simulink model "SERWO1"  (R2015b)
settings: Solver=ode1  StartTime=0.0  StopTime=Inf  FixedStep=0.001  RelTol=1e-3
PostLoadFcn:
  | , if any(exist('dsrtsu_mdlpostloadfcn', 'file') == [2, 3, 6]), try dsrtsu_mdlpostloadfcn('Execute', bdroot); catch fprintf('Error in PostLoadFcn (dsrtsu_mdlpostloadfcn) for model "%s":\n %s\n', bdroot, lasterr); end, end,
libraries: simulink x12, rtilib1104 x9
settings Model: DSRTSU_INTERNAL_RTI_VER=460  DSRTSU_INTERNAL_RTI_TYPE=rti1104  DSRTSU_INTERNAL_RTIFPGA=50  Creator=k16p800b  LastModifiedBy=lukas
settings DataIOCC: SaveFormat=Array
settings OptimizationCC: BlockReduction=off  OptimizeBlockIOStorage=off  BufferReuse=off  GlobalBufferReuse=off  ExpressionFolding=off  LocalBlockOutputs=off
settings HardwareCC: ProdBitPerPointer=32  ProdLargestAtomicFloat=None  ProdEndianess=BigEndian  ProdWordSize=32  ProdHWDeviceType=Generic->Custom  TargetIntDivRoundTo=Zero  TargetEndianess=BigEndian  TargetHWDeviceType=Generic->Custom
settings RTWCC: SystemTargetFile=rti1104.tlc  MakeCommand=make_rti  TemplateMakefile=rti1104.tmf  Description=dSPACE DS1104 Hardware Platform
settings STFCustomTargetCC: ParMdlRefBuildCompliant=on  ConcurrentExecutionCompliant=off  CPPClassGenCompliant=off  SystemTargetFile=rti1104.tlc
settings GRTTargetCC: CompOptLevelCompliant=off  ConcurrentExecutionCompliant=off  GeneratePreprocessorConditionals=Disable all  CombineOutputUpdateFcns=off  MatFileLogging=off  CPPClassGenCompliant=off  GRTInterface=on  UseToolchainInfoCompliant=off  ExtModeMexFile=noextcomm
settings ConfigComp: CovModelRefEnable=Off

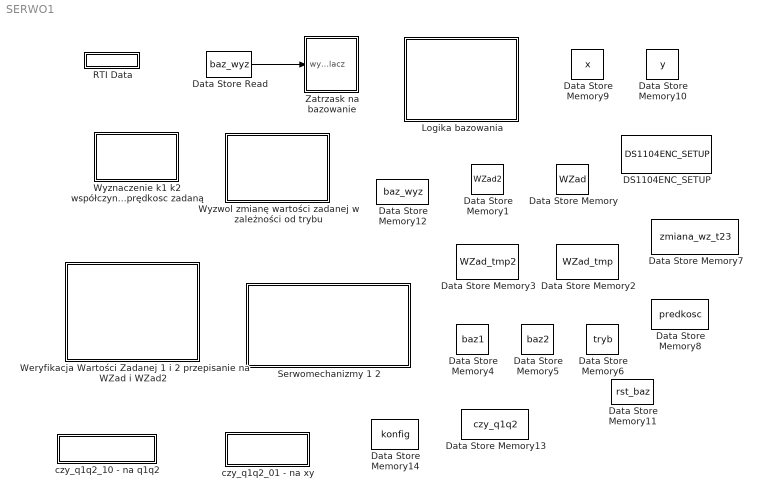
== system SERWO1 ==
  DS1104ENC_SETUP : rtilib1104/DS1104 MASTER PPC/DS1104ENC_SETUP  Reserved1=[]  Reserved2=[]  Reserved3=[]  Reserved4=[]  DialogFcn=gui1104enc_setup  UnitName={'DS1104ENC_SETUP'}  UnitValues={ [] }  DSProperties=struct('RTI',struct('Version',uint32(1),'BlockType',struct('isSLSource',uint8(0),'isSLSink',uint8(0),'isHWSource',uint8(0),'isHWSink',uint8(0),'isSetup',uint8(0),'isInline',uint8(1),'isNonInline',uint8(0),'isInterrupt',uint8(0),'isChannelwise',uint8(0)),'IOBoardType','DS1104MASTER','UnitType','ENC','Identifier','ENCSETUP','DialogType','ML','BlockSet','NONE','SlaveProcessor','NONE'))
      settings: SignalType=[0 0]
  Data Store Memory : DataStoreMemory  DataStoreName=WZad  ReadBeforeWriteMsg=warning  WriteAfterWriteMsg=warning  WriteAfterReadMsg=warning
      settings: RTWStateStorageClass=ExportedGlobal
  Data Store Memory1 : DataStoreMemory  DataStoreName=WZad2  ReadBeforeWriteMsg=warning  WriteAfterWriteMsg=warning  WriteAfterReadMsg=warning
      settings: RTWStateStorageClass=ExportedGlobal
  Data Store Memory10 : DataStoreMemory  DataStoreName=y  ReadBeforeWriteMsg=warning  WriteAfterWriteMsg=warning  WriteAfterReadMsg=warning
  Data Store Memory11 : DataStoreMemory  DataStoreName=rst_baz  ReadBeforeWriteMsg=warning  WriteAfterWriteMsg=warning  WriteAfterReadMsg=warning
  Data Store Memory12 : DataStoreMemory  DataStoreName=baz_wyz  ReadBeforeWriteMsg=warning  WriteAfterWriteMsg=warning  WriteAfterReadMsg=warning
  Data Store Memory13 : DataStoreMemory  DataStoreName=czy_q1q2  ReadBeforeWriteMsg=warning  WriteAfterWriteMsg=warning  WriteAfterReadMsg=warning
  Data Store Memory14 : DataStoreMemory  DataStoreName=konfig  ReadBeforeWriteMsg=warning  WriteAfterWriteMsg=warning  WriteAfterReadMsg=warning
  Data Store Memory2 : DataStoreMemory  DataStoreName=WZad_tmp  ReadBeforeWriteMsg=warning  WriteAfterWriteMsg=warning  WriteAfterReadMsg=warning
      settings: RTWStateStorageClass=ExportedGlobal
  Data Store Memory3 : DataStoreMemory  DataStoreName=WZad_tmp2  ReadBeforeWriteMsg=warning  WriteAfterWriteMsg=warning  WriteAfterReadMsg=warning
      settings: RTWStateStorageClass=ExportedGlobal
  Data Store Memory4 : DataStoreMemory  DataStoreName=baz1  ReadBeforeWriteMsg=warning  WriteAfterWriteMsg=warning  WriteAfterReadMsg=warning
      settings: RTWStateStorageClass=ExportedGlobal
  Data Store Memory5 : DataStoreMemory  DataStoreName=baz2  ReadBeforeWriteMsg=warning  WriteAfterWriteMsg=warning  WriteAfterReadMsg=warning
      settings: RTWStateStorageClass=ExportedGlobal
  Data Store Memory6 : DataStoreMemory  DataStoreName=tryb  ReadBeforeWriteMsg=warning  WriteAfterWriteMsg=warning  WriteAfterReadMsg=warning
      settings: RTWStateStorageClass=ExportedGlobal
  Data Store Memory7 : DataStoreMemory  DataStoreName=zmiana_wz_t23  ReadBeforeWriteMsg=warning  WriteAfterWriteMsg=warning  WriteAfterReadMsg=warning
      settings: RTWStateStorageClass=ExportedGlobal
  Data Store Memory8 : DataStoreMemory  DataStoreName=predkosc  ReadBeforeWriteMsg=warning  WriteAfterWriteMsg=warning  WriteAfterReadMsg=warning
      settings: RTWStateStorageClass=ExportedGlobal
  Data Store Memory9 : DataStoreMemory  DataStoreName=x  ReadBeforeWriteMsg=warning  WriteAfterWriteMsg=warning  WriteAfterReadMsg=warning
  Data Store Read : DataStoreRead  DataStoreName=baz_wyz
  Logika bazowania : Subsystem
      mask Display:
      | patch([0 .5 1], [0 1 0], [1 0 0])
      | fprintf('\nLogika')
      | fprintf('\n\n\n\nBazowania')
  RTI Data : Subsystem  Tag=struct('RTIDataServer',struct('RTIDataServerVs','2','RTIModelDescription','struct(''main'',''SERWO1'',''sub'','''',''isMp'',0)'))  LoadFcn="if exist('rtidc'), try,  rtidc('DataHostBlockClbLoad', gcbh); catch, disp(['Warning: ''LoadFcn'' for RTI Data block failed: ' lasterr]); end, end,"  mask(RTI_DATA_HOST){}
      mask help:
      | RTI Data Block.
      | This block is used by RTI to store internal model-dependent data.
      | Please keep this block on the root level of the model. Deleting this block will result in data loss.
      |
      | NEVER DELETE OR COPY THIS BLOCK!
      settings: CopyFcn="if exist('rtidc'), try,  rtidc('DataHostBlockClbCopy', gcbh); catch, disp(['Warning: ''CopyFcn'' for RTI Data block failed: ' lasterr]); end, end,"  DeleteFcn="if exist('rtidc'), try,  rtidc('DataHostBlockClbDelete', gcbh); catch, disp(['Warning: ''DeleteFcn'' for RTI Data block failed: ' lasterr]); end, end,"  ModelCloseFcn="if exist('rtidc'), try,  rtidc('DataHostBlockClbModelClose', gcbh); catch, disp(['Warning: ''ModelCloseFcn'' for RTI Data block failed: ' lasterr]); end, end,"  PreSaveFcn="if exist('rtidc'), try,  rtidc('DataHostBlockClbPreSave', gcbh); catch, disp(['Warning: ''PreSaveFcn'' for RTI Data block failed: ' lasterr]); end, end,"  PostSaveFcn="if exist('rtidc'), try,  rtidc('DataHostBlockClbPostSave', gcbh); catch, disp(['Warning: ''PostSaveFcn'' for RTI Data block failed: ' lasterr]); end, end,"  NameChangeFcn="if exist('rtidc'), try,  rtidc('DataHostBlockClbNameChange', gcbh); catch, disp(['Warning: ''NameChangeFcn'' for RTI Data block failed: ' lasterr]); end, end,"
      mask Help:
      | RTI Data Block.
      | This block is used by RTI to store internal model-dependent data.
      | Please keep this block on the root level of the model. Deleting this block will result in data loss.
      | 
      | NEVER DELETE OR COPY THIS BLOCK!
      mask Display:
      | text(0.5, 0.5, 'RTI Data', 'HorizontalAlignment', 'center');
      | plot([1 0]);
  Serwomechanizmy 1 2 : Subsystem
      mask Display: patch([0 .1 .9 1],[0 1  1 0],[0 0 1 ])
  Weryfikacja Wartości Zadanej 1 i 2 przepisanie na WZad i WZad2 : Subsystem
      mask Display:
      | patch([0 .5 1],[.5 1 .5],[0 1 0])
      | fprintf('\n\nWeryfikacja 1')
  Wyznaczenie k1 k2 współczynników koordynacji pomnożonych przez prędkosc zadaną : Subsystem
      mask Display: patch([0 .5 1],[1 0 1],[0 0 1])
  Wyzwol zmianę wartości zadanej w zależności od trybu : Subsystem
      mask Display: patch([0 .5 1],[1 0 1],[0 1 0])
  Zatrzask na bazowanie : Subsystem
  czy_q1q2_01 - na xy : Subsystem
  czy_q1q2_10 - na q1q2 : Subsystem
  wires:
  Data Store Read/1 -> Zatrzask na bazowanie/1(wyzwalacz)

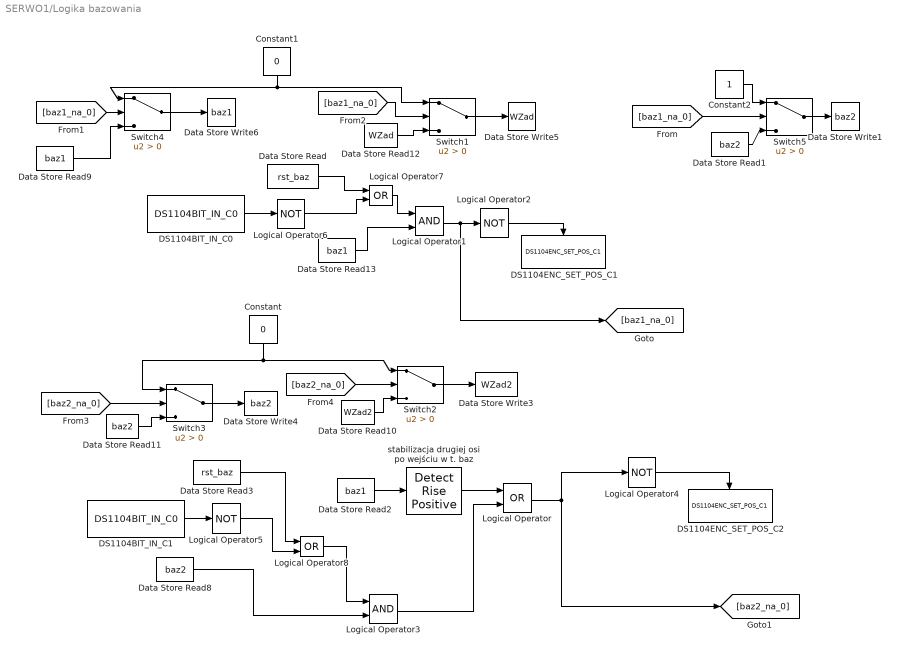
== system SERWO1/Logika bazowania ==
  Constant : Constant  Value=0
  Constant1 : Constant  Value=0
  Constant2 : Constant
  DS1104BIT_IN_C0 : rtilib1104/DS1104 MASTER PPC/DS1104BIT_IN_C0  ChannelNo=0  Reserved1=[]  Reserved2=[]  Reserved3=[]  Reserved4=[]  DialogFcn=gui1104bit_in  UnitName={'DS1104BIT_IN_C'}  UnitValues={ 0 }  DSProperties=struct('RTI',struct('Version',uint32(1),'BlockType',struct('isSLSource',uint8(1),'isSLSink',uint8(0),'isHWSource',uint8(1),'isHWSink',uint8(0),'isSetup',uint8(0),'isInline',uint8(1),'isNonInline',uint8(0),'isInterrupt',uint8(0),'isChannelwise',uint8(1)),'IOBoardType','DS1104MASTER','UnitType','BIT','Identifier','BITINCH','DialogType','ML','BlockSet','NONE','SlaveProcessor','NONE'))
  DS1104BIT_IN_C1 : rtilib1104/DS1104 MASTER PPC/DS1104BIT_IN_C0  ChannelNo=1  Reserved1=[]  Reserved2=[]  Reserved3=[]  Reserved4=[]  DialogFcn=gui1104bit_in  UnitName={'DS1104BIT_IN_C'}  UnitValues={1}  DSProperties=struct('RTI',struct('Version',uint32(1),'BlockType',struct('isSLSource',uint8(1),'isSLSink',uint8(0),'isHWSource',uint8(1),'isHWSink',uint8(0),'isSetup',uint8(0),'isInline',uint8(1),'isNonInline',uint8(0),'isInterrupt',uint8(0),'isChannelwise',uint8(1)),'IOBoardType','DS1104MASTER','UnitType','BIT','Identifier','BITINCH','DialogType','ML','BlockSet','NONE','SlaveProcessor','NONE'))
  DS1104ENC_SET_POS_C1 : rtilib1104/DS1104 MASTER PPC/DS1104ENC_SET_POS_C1  ChannelNo=1  PosValue=0  Reserved1=[]  Reserved2=[]  Reserved3=[]  Reserved4=[]  DialogFcn=gui1104enc_set_pos  UnitName={'DS1104ENC_SET_POS_C'}  UnitValues={ 1 }  DSProperties=struct('RTI',struct('Version',uint32(1),'BlockType',struct('isSLSource',uint8(0),'isSLSink',uint8(1),'isHWSource',uint8(0),'isHWSink',uint8(1),'isSetup',uint8(0),'isInline',uint8(1),'isNonInline',uint8(0),'isInterrupt',uint8(0),'isChannelwise',uint8(1)),'IOBoardType','DS1104MASTER','UnitType','ENC','Identifier','ENCRESET','DialogType','ML','BlockSet','NONE','SlaveProcessor','NONE'))
  DS1104ENC_SET_POS_C2 : rtilib1104/DS1104 MASTER PPC/DS1104ENC_SET_POS_C1  ChannelNo=2  PosValue=0  Reserved1=[]  Reserved2=[]  Reserved3=[]  Reserved4=[]  DialogFcn=gui1104enc_set_pos  UnitName={'DS1104ENC_SET_POS_C'}  UnitValues={2}  DSProperties=struct('RTI',struct('Version',uint32(1),'BlockType',struct('isSLSource',uint8(0),'isSLSink',uint8(1),'isHWSource',uint8(0),'isHWSink',uint8(1),'isSetup',uint8(0),'isInline',uint8(1),'isNonInline',uint8(0),'isInterrupt',uint8(0),'isChannelwise',uint8(1)),'IOBoardType','DS1104MASTER','UnitType','ENC','Identifier','ENCRESET','DialogType','ML','BlockSet','NONE','SlaveProcessor','NONE'))
  Data Store Read : DataStoreRead  DataStoreName=rst_baz
  Data Store Read1 : DataStoreRead  DataStoreName=baz2
  Data Store Read10 : DataStoreRead  DataStoreName=WZad2
  Data Store Read11 : DataStoreRead  DataStoreName=baz2
  Data Store Read12 : DataStoreRead  DataStoreName=WZad
  Data Store Read13 : DataStoreRead  DataStoreName=baz1
  Data Store Read2 : DataStoreRead  DataStoreName=baz1
  Data Store Read3 : DataStoreRead  DataStoreName=rst_baz
  Data Store Read8 : DataStoreRead  DataStoreName=baz2
  Data Store Read9 : DataStoreRead  DataStoreName=baz1
  Data Store Write1 : DataStoreWrite  DataStoreName=baz2
  Data Store Write3 : DataStoreWrite  DataStoreName=WZad2
  Data Store Write4 : DataStoreWrite  DataStoreName=baz2
  Data Store Write5 : DataStoreWrite  DataStoreName=WZad
  Data Store Write6 : DataStoreWrite  DataStoreName=baz1
  Logical Operator : Logic  Operator=OR  AllPortsSameDT=off  OutDataTypeStr=boolean
  Logical Operator1 : Logic  AllPortsSameDT=off  OutDataTypeStr=boolean
  Logical Operator{2,4..6} (4 alike) : Logic  Operator=NOT  AllPortsSameDT=off  OutDataTypeStr=boolean
  Logical Operator3 : Logic  AllPortsSameDT=off  OutDataTypeStr=boolean
  Logical Operator7 : Logic  Operator=OR  AllPortsSameDT=off  OutDataTypeStr=boolean
  Logical Operator8 : Logic  Operator=OR  AllPortsSameDT=off  OutDataTypeStr=boolean
  Switch{1..5} (5 alike) : Switch  Criteria=u2 > Threshold
  stabilizacja drugiej osi po wejściu w t. baz : simulink/Logic and Bit Operations/Detect Rise Positive  vinit=0  InputProcessing=Inherited  OutDataTypeStr=boolean
  wires:
  DS1104BIT_IN_C1/1 -> Logical Operator5/1
  Logical Operator4/1 -> DS1104ENC_SET_POS_C2/Trigger
  Data Store Read8/1 -> Logical Operator3/2
  Switch3/1 -> Data Store Write4/1
  Switch2/1 -> Data Store Write3/1
  DS1104BIT_IN_C0/1 -> Logical Operator6/1
  Data Store Read9/1 -> Switch4/3
  Data Store Read13/1 -> Logical Operator1/2
  Data Store Read12/1 -> Switch1/3
  Data Store Read10/1 -> Switch2/3
  Switch4/1 -> Data Store Write6/1
  Switch1/1 -> Data Store Write5/1
  Constant1/1 -> Switch1/1, Switch4/1
  Constant/1 -> Switch2/1, Switch3/1
  Data Store Read11/1 -> Switch3/3
  Constant2/1 -> Switch5/1
  Data Store Read1/1 -> Switch5/3
  Switch5/1 -> Data Store Write1/1
  [baz1_na_0] -> Switch5/2
  [baz1_na_0] -> Switch4/2
  [baz1_na_0] -> Switch1/2
  [baz2_na_0] -> Switch3/2
  [baz2_na_0] -> Switch2/2
  Data Store Read2/1 -> stabilizacja drugiej osi po wejściu w t. baz/1
  stabilizacja drugiej osi po wejściu w t. baz/1 -> Logical Operator/1
  Data Store Read/1 -> Logical Operator7/1
  Logical Operator5/1 -> Logical Operator8/2
  Data Store Read3/1 -> Logical Operator8/1
  Logical Operator1/1 -> [baz1_na_0], Logical Operator2/1
  Logical Operator/1 -> [baz2_na_0], Logical Operator4/1
  Logical Operator2/1 -> DS1104ENC_SET_POS_C1/Trigger
  Logical Operator6/1 -> Logical Operator7/2
  Logical Operator7/1 -> Logical Operator1/1
  Logical Operator8/1 -> Logical Operator3/1
  Logical Operator3/1 -> Logical Operator/2

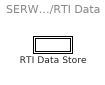
== system SERWO1/RTI Data ==
  RTI Data Store : Subsystem  Tag="struct('private',struct('version',struct('dsVer',uint32(2),'dsVerCreation',uint32(2),'RTI',struct('ver','7.4','type','RTI1104')),'access',struct('type','Model','isPerm',1,'created',['07-Mar-2016 08:19:13'],'modified',['21-Mar-2016 09:28:19'],'location','')),'public',struct('main',struct('data',[]),'sub',struct('name',{{'SERWO1'}},'data',{{struct('TH',struct('thTaskInfo',struct('taskType',{'TIMER','HWINT','TMRINT','SWINT','GLINT'},'tasksNumOf',{1,0,0,0,0},'srcIds',{{'TIMERA'},{},{},{},{}},'taskNames',{{['Timer Task 1']},{},{},{},{}})),'th_tc',struct('dataType','TASK','taskGroupId','','taskGroupList',{{}},'taskSchedulingPolicy','FCFS','taskType','TIMER','blkh',-1,'srcId','TIMERA','srcSgnName',['Timer A interrupt'],'srcCpuName','','taskName',['Timer Task 1  [0.001] s'],'taskNameDisplayExt','','smplTime',0.001,'smplTimeOffs',0,'hasFixedPriority',0,'priority',1,'hasFixedOvc',0,'ovcType',1,'ovcMax',1),'tc_th',struct('dataType','TASK','taskGroupId','','taskGroupList',{{}},'taskSchedulingPolicy','FCFS','taskType','TIMER','blkh',-1,'srcId','TIMERA','srcSgnName',['Timer A interrupt'],'srcCpuName','','taskName',['Timer Task 1  [0.001] s'],'taskNameDisplayExt','','smplTime',0.001,'smplTimeOffs',0,'hasFixedPriority',0,'priority',1,'hasFixedOvc',0,'ovcType',1,'ovcMax',1))}})))"  mask(RTI_DATA_STORE){}
      mask help:
      | RTI Data Store Block. This block is used by RTI to store internal model dependent data. Deleting this block will result in data loss.
      |
      | NEVER DELETE, COPY, OR MODIFY THIS BLOCK!
      mask Help:
      | RTI Data Store Block. This block is used by RTI to store internal model dependent data. Deleting this block will result in data loss.
      | 
      | NEVER DELETE, COPY, OR MODIFY THIS BLOCK!
      mask Display: text(0.5, 0.5, ' ', 'HorizontalAlignment', 'center');

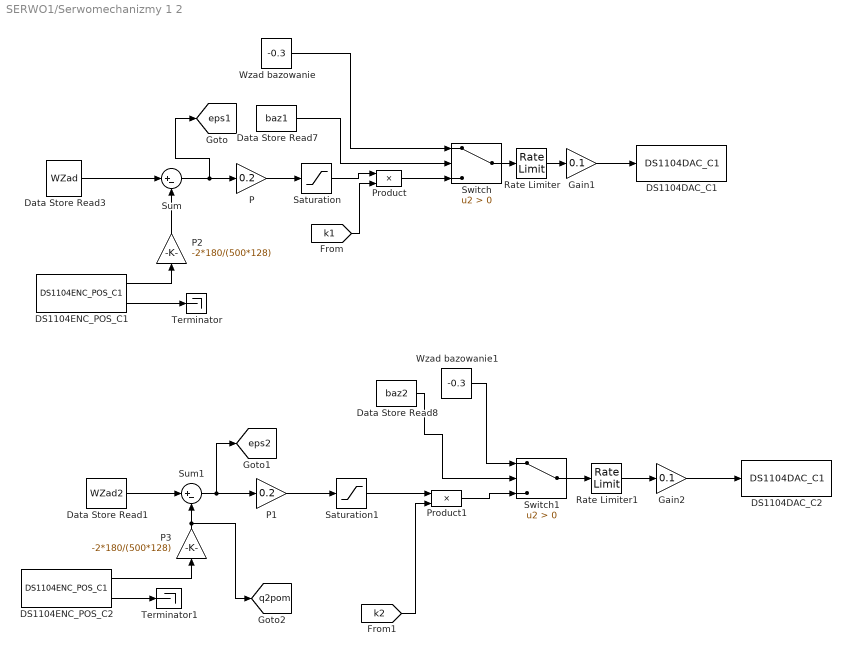
== system SERWO1/Serwomechanizmy 1 2 ==
  DS1104DAC_C1 : rtilib1104/DS1104 MASTER PPC/DS1104DAC_C1  ChannelNo=1  InitValue=0  TermMode=1  TermValue=0  Reserved1=[]  Reserved2=[]  Reserved3=[]  Reserved4=[]  DialogFcn=gui1104dac  UnitName={ 'DS1104DAC_C'}  UnitValues={ 1 }  DSProperties=struct('RTI',struct('Version',uint32(1),'BlockType',struct('isSLSource',uint8(0),'isSLSink',uint8(1),'isHWSource',uint8(0),'isHWSink',uint8(1),'isSetup',uint8(0),'isInline',uint8(1),'isNonInline',uint8(0),'isInterrupt',uint8(0),'isChannelwise',uint8(1)),'IOBoardType','DS1104MASTER','UnitType','DAC','Identifier','DAC','DialogType','ML','BlockSet','NONE','SlaveProcessor','NONE'))
  DS1104DAC_C2 : rtilib1104/DS1104 MASTER PPC/DS1104DAC_C1  ChannelNo=2  InitValue=0  TermMode=1  TermValue=0  Reserved1=[]  Reserved2=[]  Reserved3=[]  Reserved4=[]  DialogFcn=gui1104dac  UnitName={ 'DS1104DAC_C'}  UnitValues={ 2 }  DSProperties=struct('RTI',struct('Version',uint32(1),'BlockType',struct('isSLSource',uint8(0),'isSLSink',uint8(1),'isHWSource',uint8(0),'isHWSink',uint8(1),'isSetup',uint8(0),'isInline',uint8(1),'isNonInline',uint8(0),'isInterrupt',uint8(0),'isChannelwise',uint8(1)),'IOBoardType','DS1104MASTER','UnitType','DAC','Identifier','DAC','DialogType','ML','BlockSet','NONE','SlaveProcessor','NONE'))
  DS1104ENC_POS_C1 : rtilib1104/DS1104 MASTER PPC/DS1104ENC_POS_C1  ChannelNo=1  PosValue=0  Reserved1=[]  Reserved2=[]  Reserved3=[]  Reserved4=[]  DialogFcn=gui1104enc_pos  UnitName={'DS1104ENC_POS_C'}  UnitValues={ 1 }  DSProperties=struct('RTI',struct('Version',uint32(1),'BlockType',struct('isSLSource',uint8(1),'isSLSink',uint8(0),'isHWSource',uint8(1),'isHWSink',uint8(0),'isSetup',uint8(0),'isInline',uint8(1),'isNonInline',uint8(0),'isInterrupt',uint8(0),'isChannelwise',uint8(1)),'IOBoardType','DS1104MASTER','UnitType','ENC','Identifier','ENCPOSCH','DialogType','ML','BlockSet','NONE','SlaveProcessor','NONE'))
  DS1104ENC_POS_C2 : rtilib1104/DS1104 MASTER PPC/DS1104ENC_POS_C1  ChannelNo=2  PosValue=0  Reserved1=[]  Reserved2=[]  Reserved3=[]  Reserved4=[]  DialogFcn=gui1104enc_pos  UnitName={'DS1104ENC_POS_C'}  UnitValues={2}  DSProperties=struct('RTI',struct('Version',uint32(1),'BlockType',struct('isSLSource',uint8(1),'isSLSink',uint8(0),'isHWSource',uint8(1),'isHWSink',uint8(0),'isSetup',uint8(0),'isInline',uint8(1),'isNonInline',uint8(0),'isInterrupt',uint8(0),'isChannelwise',uint8(1)),'IOBoardType','DS1104MASTER','UnitType','ENC','Identifier','ENCPOSCH','DialogType','ML','BlockSet','NONE','SlaveProcessor','NONE'))
  Data Store Read1 : DataStoreRead  DataStoreName=WZad2
  Data Store Read3 : DataStoreRead  DataStoreName=WZad
  Data Store Read7 : DataStoreRead  DataStoreName=baz1
  Data Store Read8 : DataStoreRead  DataStoreName=baz2
  Gain1 : Gain  Gain=0.1
  Gain2 : Gain  Gain=0.1
  P : Gain  Gain=0.2
  P1 : Gain  Gain=0.2
  P2 : Gain  Gain=-2*180/(500*128)
  P3 : Gain  Gain=-2*180/(500*128)
  Product : Product
  Product1 : Product
  Rate Limiter : RateLimiter  RisingSlewLimit=50  FallingSlewLimit=-50  SampleTimeMode=inherited
  Rate Limiter1 : RateLimiter  RisingSlewLimit=50  FallingSlewLimit=-50  SampleTimeMode=inherited
  Saturation : Saturate  UpperLimit=3  LowerLimit=-3
  Saturation1 : Saturate  UpperLimit=3  LowerLimit=-3
  Sum : Sum  Inputs=|+-
  Sum1 : Sum  Inputs=|+-
  Switch : Switch  Criteria=u2 > Threshold
  Switch1 : Switch  Criteria=u2 > Threshold
  Terminator : Terminator
  Terminator1 : Terminator
  Wzad bazowanie : Constant  Value=-0.3
  Wzad bazowanie1 : Constant  Value=-0.3
  tag scope: eps1=global, eps2=global, q2pom=global
  wires:
  Saturation1/1 -> Product1/1
  [k1] -> Product/2
  Product/1 -> Switch/3
  Saturation/1 -> Product/1
  Product1/1 -> Switch1/3
  Sum/1 -> [eps1], P/1
  P/1 -> Saturation/1
  Rate Limiter/1 -> Gain1/1
  Gain1/1 -> DS1104DAC_C1/1
  Data Store Read1/1 -> Sum1/1
  Sum1/1 -> [eps2], P1/1
  P1/1 -> Saturation1/1
  Rate Limiter1/1 -> Gain2/1
  Gain2/1 -> DS1104DAC_C2/1
  DS1104ENC_POS_C1/1 -> P2/1
  P2/1 -> Sum/2
  DS1104ENC_POS_C2/1 -> P3/1
  P3/1 -> [q2pom], Sum1/2
  DS1104ENC_POS_C1/2 -> Terminator/1
  DS1104ENC_POS_C2/2 -> Terminator1/1
  Data Store Read3/1 -> Sum/1
  Switch/1 -> Rate Limiter/1
  Data Store Read7/1 -> Switch/2
  Wzad bazowanie/1 -> Switch/1
  Switch1/1 -> Rate Limiter1/1
  Data Store Read8/1 -> Switch1/2
  Wzad bazowanie1/1 -> Switch1/1
  [k2] -> Product1/2

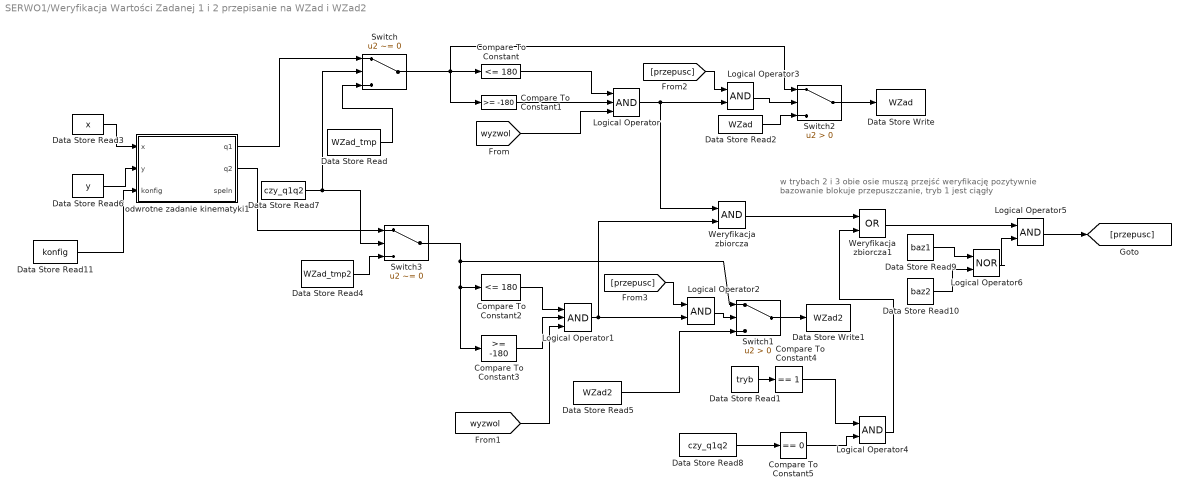
== system SERWO1/Weryfikacja Wartości Zadanej 1 i 2 przepisanie na WZad i WZad2 ==
  note: w trybach 2 i 3 obie osie muszą przejść weryfikację pozytywnie
      | bazowanie blokuje przepuszczanie, tryb 1 jest ciągły
  Compare To Constant : simulink/Logic and Bit Operations/Compare To Constant  relop=<=  const=180  OutDataTypeStr=boolean
  Compare To Constant1 : simulink/Logic and Bit Operations/Compare To Constant  relop=>=  const=-180  OutDataTypeStr=boolean
  Compare To Constant2 : simulink/Logic and Bit Operations/Compare To Constant  relop=<=  const=180  OutDataTypeStr=boolean
  Compare To Constant3 : simulink/Logic and Bit Operations/Compare To Constant  relop=>=  const=-180  OutDataTypeStr=boolean
  Compare To Constant4 : simulink/Logic and Bit Operations/Compare To Constant  relop===  const=1  OutDataTypeStr=boolean
  Compare To Constant5 : simulink/Logic and Bit Operations/Compare To Constant  relop===  const=0  OutDataTypeStr=boolean
  Data Store Read : DataStoreRead  DataStoreName=WZad_tmp
  Data Store Read1 : DataStoreRead  DataStoreName=tryb
  Data Store Read10 : DataStoreRead  DataStoreName=baz2
  Data Store Read11 : DataStoreRead  DataStoreName=konfig
  Data Store Read2 : DataStoreRead  DataStoreName=WZad
  Data Store Read3 : DataStoreRead  DataStoreName=x
  Data Store Read4 : DataStoreRead  DataStoreName=WZad_tmp2
  Data Store Read5 : DataStoreRead  DataStoreName=WZad2
  Data Store Read6 : DataStoreRead  DataStoreName=y
  Data Store Read7 : DataStoreRead  DataStoreName=czy_q1q2
  Data Store Read8 : DataStoreRead  DataStoreName=czy_q1q2
  Data Store Read9 : DataStoreRead  DataStoreName=baz1
  Data Store Write : DataStoreWrite  DataStoreName=WZad
  Data Store Write1 : DataStoreWrite  DataStoreName=WZad2
  Logical Operator : Logic  Inputs=3  AllPortsSameDT=off  OutDataTypeStr=boolean
  Logical Operator1 : Logic  Inputs=3  AllPortsSameDT=off  OutDataTypeStr=boolean
  Logical Operator{2..5} (4 alike) : Logic  AllPortsSameDT=off  OutDataTypeStr=boolean
  Logical Operator6 : Logic  Operator=NOR  AllPortsSameDT=off  OutDataTypeStr=boolean
  Switch : Switch  Criteria=u2 ~= 0  Threshold=2
  Switch1 : Switch  Criteria=u2 > Threshold
  Switch2 : Switch  Criteria=u2 > Threshold
  Switch3 : Switch  Criteria=u2 ~= 0  Threshold=2
  Weryfikacja zbiorcza : Logic  AllPortsSameDT=off  OutDataTypeStr=boolean
  Weryfikacja zbiorcza1 : Logic  Operator=OR  AllPortsSameDT=off  OutDataTypeStr=boolean
  odwrotne zadanie kinematyki1 : MATLAB Function  TreatAsAtomicUnit=on
  wires:
  Data Store Read2/1 -> Switch2/3
  Compare To Constant/1 -> Logical Operator/1
  Switch/1 -> Switch2/1, Compare To Constant/1, Compare To Constant1/1
  Compare To Constant1/1 -> Logical Operator/2
  Logical Operator/1 -> Logical Operator3/2, Weryfikacja zbiorcza/1
  Switch2/1 -> Data Store Write/1
  [wyzwol] -> Logical Operator/3
  Data Store Read5/1 -> Switch1/3
  Compare To Constant2/1 -> Logical Operator1/1
  Switch3/1 -> Compare To Constant3/1, Compare To Constant2/1, Switch1/1
  Compare To Constant3/1 -> Logical Operator1/2
  Logical Operator1/1 -> Logical Operator2/2, Weryfikacja zbiorcza/2
  Switch1/1 -> Data Store Write1/1
  [wyzwol] -> Logical Operator1/3
  Weryfikacja zbiorcza/1 -> Weryfikacja zbiorcza1/1
  [przepusc] -> Logical Operator3/1
  Logical Operator3/1 -> Switch2/2
  Logical Operator2/1 -> Switch1/2
  [przepusc] -> Logical Operator2/1
  Data Store Read3/1 -> odwrotne zadanie kinematyki1/1(x)
  Data Store Read6/1 -> odwrotne zadanie kinematyki1/2(y)
  Data Store Read7/1 -> Switch3/2, Switch/2
  odwrotne zadanie kinematyki1/1(q1) -> Switch/1
  Data Store Read/1 -> Switch/3
  odwrotne zadanie kinematyki1/2(q2) -> Switch3/1
  Data Store Read4/1 -> Switch3/3
  Weryfikacja zbiorcza1/1 -> Logical Operator5/1
  Compare To Constant5/1 -> Logical Operator4/2
  Data Store Read1/1 -> Compare To Constant4/1
  Compare To Constant4/1 -> Logical Operator4/1
  Data Store Read8/1 -> Compare To Constant5/1
  Logical Operator4/1 -> Weryfikacja zbiorcza1/2
  Data Store Read9/1 -> Logical Operator6/1
  Data Store Read10/1 -> Logical Operator6/2
  Logical Operator6/1 -> Logical Operator5/2
  Logical Operator5/1 -> [przepusc]
  Data Store Read11/1 -> odwrotne zadanie kinematyki1/3(konfig)

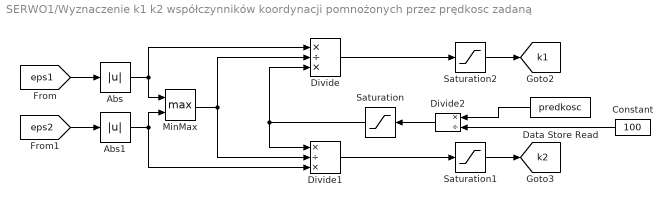
== system SERWO1/Wyznaczenie k1 k2 współczynników koordynacji pomnożonych przez prędkosc zadaną ==
  Abs : Abs
  Abs1 : Abs
  Constant : Constant  Value=100
  Data Store Read : DataStoreRead  DataStoreName=predkosc
  Divide : Product  Inputs=*/*
  Divide1 : Product  Inputs=*/*
  Divide2 : Product  Inputs=*/
  MinMax : MinMax  Function=max  Inputs=2
  Saturation : Saturate  UpperLimit=1  LowerLimit=0.1
  Saturation1 : Saturate  UpperLimit=1  LowerLimit=0.1
  Saturation2 : Saturate  UpperLimit=1  LowerLimit=0.1
  tag scope: k1=global, k2=global
  wires:
  Abs/1 -> MinMax/1, Divide/1
  [eps2] -> Abs1/1
  Abs1/1 -> Divide1/3, MinMax/2
  [eps1] -> Abs/1
  Saturation/1 -> Divide/3, Divide1/1
  MinMax/1 -> Divide1/2, Divide/2
  Saturation2/1 -> [k1]
  Saturation1/1 -> [k2]
  Divide1/1 -> Saturation1/1
  Divide/1 -> Saturation2/1
  Constant/1 -> Divide2/2
  Data Store Read/1 -> Divide2/1
  Divide2/1 -> Saturation/1

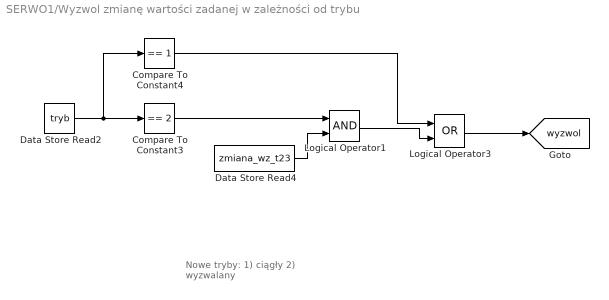
== system SERWO1/Wyzwol zmianę wartości zadanej w zależności od trybu ==
  note: Nowe tryby:
      | 1) ciągły
      | 2) wyzwalany
  Compare To Constant3 : simulink/Logic and Bit Operations/Compare To Constant  relop===  const=2  OutDataTypeStr=boolean
  Compare To Constant4 : simulink/Logic and Bit Operations/Compare To Constant  relop===  const=1  OutDataTypeStr=boolean
  Data Store Read2 : DataStoreRead  DataStoreName=tryb
  Data Store Read4 : DataStoreRead  DataStoreName=zmiana_wz_t23
  Logical Operator1 : Logic  AllPortsSameDT=off  OutDataTypeStr=boolean
  Logical Operator3 : Logic  Operator=OR  AllPortsSameDT=off  OutDataTypeStr=boolean
  tag scope: wyzwol=global
  wires:
  Logical Operator3/1 -> [wyzwol]
  Compare To Constant4/1 -> Logical Operator3/1
  Compare To Constant3/1 -> Logical Operator1/1
  Logical Operator1/1 -> Logical Operator3/2
  Data Store Read2/1 -> Compare To Constant3/1, Compare To Constant4/1
  Data Store Read4/1 -> Logical Operator1/2

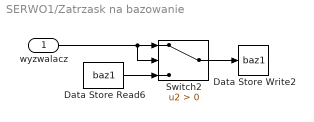
== system SERWO1/Zatrzask na bazowanie ==
  wyzwalacz : Inport
  Data Store Read6 : DataStoreRead  DataStoreName=baz1
  Data Store Write2 : DataStoreWrite  DataStoreName=baz1
  Switch2 : Switch  Criteria=u2 > Threshold
  wires:
  Data Store Read6/1 -> Switch2/3
  wyzwalacz/1 -> Switch2/2, Switch2/1
  Switch2/1 -> Data Store Write2/1

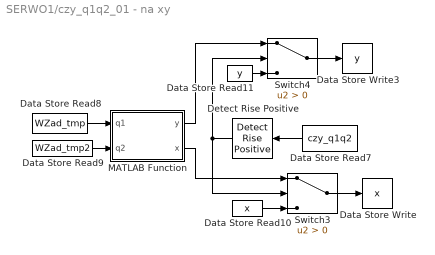
== system SERWO1/czy_q1q2_01 - na xy ==
  Data Store Read10 : DataStoreRead  DataStoreName=x
  Data Store Read11 : DataStoreRead  DataStoreName=y
  Data Store Read7 : DataStoreRead  DataStoreName=czy_q1q2
  Data Store Read8 : DataStoreRead  DataStoreName=WZad_tmp
  Data Store Read9 : DataStoreRead  DataStoreName=WZad_tmp2
  Data Store Write : DataStoreWrite  DataStoreName=x
  Data Store Write3 : DataStoreWrite  DataStoreName=y
  Detect Rise Positive : simulink/Logic and Bit Operations/Detect Rise Positive  vinit=0  InputProcessing=Inherited  OutDataTypeStr=boolean
  MATLAB Function : MATLAB Function  TreatAsAtomicUnit=on
  Switch3 : Switch  Criteria=u2 > Threshold
  Switch4 : Switch  Criteria=u2 > Threshold
  wires:
  Data Store Read7/1 -> Detect Rise Positive/1
  MATLAB Function/2(x) -> Switch3/1
  Data Store Read8/1 -> MATLAB Function/1(q1)
  Data Store Read9/1 -> MATLAB Function/2(q2)
  Switch3/1 -> Data Store Write/1
  Data Store Read10/1 -> Switch3/3
  Detect Rise Positive/1 -> Switch4/2, Switch3/2
  MATLAB Function/1(y) -> Switch4/1
  Switch4/1 -> Data Store Write3/1
  Data Store Read11/1 -> Switch4/3

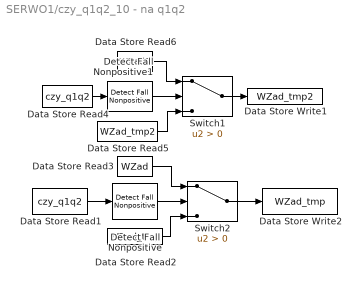
== system SERWO1/czy_q1q2_10 - na q1q2 ==
  Data Store Read1 : DataStoreRead  DataStoreName=czy_q1q2
  Data Store Read2 : DataStoreRead  DataStoreName=WZad_tmp
  Data Store Read3 : DataStoreRead  DataStoreName=WZad
  Data Store Read4 : DataStoreRead  DataStoreName=czy_q1q2
  Data Store Read5 : DataStoreRead  DataStoreName=WZad_tmp2
  Data Store Read6 : DataStoreRead  DataStoreName=WZad2
  Data Store Write1 : DataStoreWrite  DataStoreName=WZad_tmp2
  Data Store Write2 : DataStoreWrite  DataStoreName=WZad_tmp
  Detect Fall Nonpositive : simulink/Logic and Bit Operations/Detect Fall Nonpositive  vinit=0  InputProcessing=Inherited  OutDataTypeStr=boolean
  Detect Fall Nonpositive1 : simulink/Logic and Bit Operations/Detect Fall Nonpositive  vinit=0  InputProcessing=Inherited  OutDataTypeStr=boolean
  Switch1 : Switch  Criteria=u2 > Threshold
  Switch2 : Switch  Criteria=u2 > Threshold
  wires:
  Data Store Read2/1 -> Switch2/3
  Data Store Read1/1 -> Detect Fall Nonpositive/1
  Data Store Read3/1 -> Switch2/1
  Switch2/1 -> Data Store Write2/1
  Switch1/1 -> Data Store Write1/1
  Data Store Read4/1 -> Detect Fall Nonpositive1/1
  Detect Fall Nonpositive1/1 -> Switch1/2
  Data Store Read6/1 -> Switch1/1
  Data Store Read5/1 -> Switch1/3
  Detect Fall Nonpositive/1 -> Switch2/2

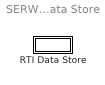
== system SERWO1/RTI Data/RTI Data Store ==
  RTI Data Store : Subsystem  mask(RTI_DATA_STORE){}
      mask help:
      | RTI Data Store Block. This block is used by RTI to store internal model dependent data. Deleting this block will result in data loss.
      |
      | NEVER DELETE, COPY, OR MODIFY THIS BLOCK!
      mask Help:
      | RTI Data Store Block. This block is used by RTI to store internal model dependent data. Deleting this block will result in data loss.
      | 
      | NEVER DELETE, COPY, OR MODIFY THIS BLOCK!
      mask Display: text(0.5, 0.5, ' ', 'HorizontalAlignment', 'center');

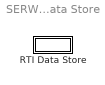
== system SERWO1/RTI Data/RTI Data Store/RTI Data Store ==
  RTI Data Store : Subsystem  mask(RTI_DATA_STORE){}
      mask help:
      | RTI Data Store Block. This block is used by RTI to store internal model dependent data. Deleting this block will result in data loss.
      |
      | NEVER DELETE, COPY, OR MODIFY THIS BLOCK!
      mask Help:
      | RTI Data Store Block. This block is used by RTI to store internal model dependent data. Deleting this block will result in data loss.
      | 
      | NEVER DELETE, COPY, OR MODIFY THIS BLOCK!
      mask Display: text(0.5, 0.5, ' ', 'HorizontalAlignment', 'center');

== system SERWO1/RTI Data/RTI Data Store/RTI Data Store/RTI Data Store ==
  RTI Data Store : Subsystem  mask(RTI_DATA_STORE){}
      mask help:
      | RTI Data Store Block. This block is used by RTI to store internal model dependent data. Deleting this block will result in data loss.
      |
      | NEVER DELETE, COPY, OR MODIFY THIS BLOCK!
      mask Help:
      | RTI Data Store Block. This block is used by RTI to store internal model dependent data. Deleting this block will result in data loss.
      | 
      | NEVER DELETE, COPY, OR MODIFY THIS BLOCK!
      mask Display: text(0.5, 0.5, ' ', 'HorizontalAlignment', 'center');

== system SERWO1/RTI Data/RTI Data Store/RTI Data Store/RTI Data Store/RTI Data Store ==

== matlab function SERWO1/Weryfikacja Wartości Zadanej 1 i 2 przepisanie na WZad i WZad2/odwrotne zadanie kinematyki1 ==
  data: x input; y input; q1 output; q2 output; speln output; konfig input
function [q1,q2,speln] = fcn(x,y,konfig)
%#codegen
R1 = 630;
R2 = 510;
R = sqrt(x.^2 + y.^2);
if R^2<(R1+R2)^2 && R^2 > (R1-R2)^2
    speln = 1;
    L = (R1.^2 + R2.^2 - R.^2)./(2*R1*R2);
    q2 = atan2(sqrt(1-L^2),L);
    if konfig==1
        q2=-q2;
    end
    q1 = atan2(y,x) - atan(R2*sin(q2)/(R1-R2*cos(q2)));
    
    q1 = q1*180/pi;
    q2 = q2*180/pi;
    if q1<-180
        q1=q1+360;
    elseif q1>180
        q1=q1-360;
    end
    if q2<-180
        q2=q2+360;
    elseif q2>180
        q2=q2-360;
    end
else
    speln=0;
    q1=200;
    q2=200;
end

== matlab function SERWO1/czy_q1q2_01 - na xy/MATLAB Function ==
  data: y output; x output; q1 input; q2 input
function [y,x] = fcn(q1,q2)
%#codegen
q1 = pi/180*q1;
q2 = pi/180*q2;
R1 = 630;
R2 = 510;
y = R1*sin(q1)+R2*sin(q2-q1);
x = R1*cos(q1)-R2*cos(q2-q1);
